simulink model "Three_Phase_180_VSI"  (R2023b)
settings: Solver=VariableStepAuto  StartTime=0.0  StopTime=0.1  RelTol=1e-3
libraries: spsDiodeLib x6, spsIGBTLib x6, spsVoltageMeasurementLib x6, spsSeriesRLCBranchLib x3, spsDCVoltageSourceLib x2, spspowerguiLib x1
settings Model: Creator=prita  LastModifiedBy=KULDIP
settings DebuggingCC: UnconnectedInputMsg=warning  UnconnectedOutputMsg=warning  UnconnectedLineMsg=warning
settings ModelReferenceCC: EnableRefExpFcnMdlSchedulingChecks=on
settings RTWCC: DLArmComputeVersion=19.05

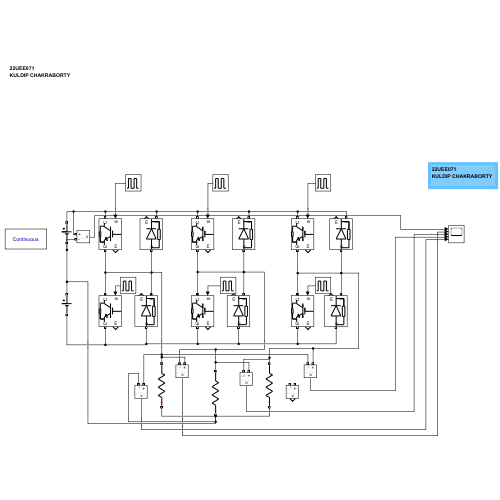
[thumbnail: Simulink's stored preview of the top-level diagram]
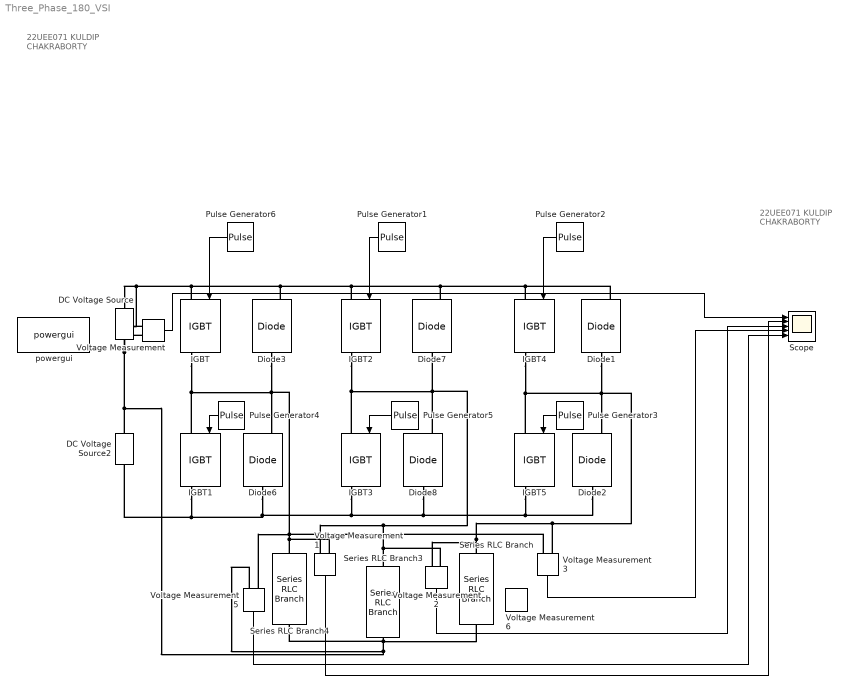
== system Three_Phase_180_VSI ==
  note: 22UEE071
      | KULDIP CHAKRABORTY
  note: 22UEE071
      | KULDIP CHAKRABORTY
  DC Voltage Source : spsDCVoltageSourceLib/DC Voltage Source  Amplitude=25  Measurements=None
  DC Voltage Source2 : spsDCVoltageSourceLib/DC Voltage Source  Amplitude=25  Measurements=None
  Diode{1..3,6..8} (6 alike) : spsDiodeLib/Diode  Ron=0.001  Lon=0  Vf=0.8  IC=0  UseSnubber=0  Rs=500  Cs=250e-9  Measurements=on
  IGBT{,1..5} (6 alike) : spsIGBTLib/IGBT  Ron=0.001  Lon=0  Vf=0  Tf=1e-6  Tt=2e-6  IC=0  Rs=1e5  Cs=inf  Measurements=on
  Pulse Generator1 : DiscretePulseGenerator  PulseType=Time based  Period=0.02  PulseWidth=50  PhaseDelay=(0.02/360)*120
  Pulse Generator2 : DiscretePulseGenerator  PulseType=Time based  Period=0.02  PulseWidth=50  PhaseDelay=(0.02/360)*240
  Pulse Generator3 : DiscretePulseGenerator  PulseType=Time based  Period=0.02  PulseWidth=50  PhaseDelay=(0.02/360)*420
  Pulse Generator4 : DiscretePulseGenerator  PulseType=Time based  Period=0.02  PulseWidth=50  PhaseDelay=(0.02/360)*180
  Pulse Generator5 : DiscretePulseGenerator  PulseType=Time based  Period=0.02  PulseWidth=50  PhaseDelay=(0.02/360)*300
  Pulse Generator6 : DiscretePulseGenerator  PulseType=Time based  Period=0.02  PulseWidth=50
  Scope : Scope  NumInputPorts=5
  Series RLC Branch : spsSeriesRLCBranchLib/Series RLC Branch  LConnTagsString=__new0  RConnTagsString=__new0  BranchType=R  Resistance=1  Inductance=1e-3  SetiL0=off  InitialCurrent=0  Capacitance=1e-6  Setx0=off  InitialVoltage=0  Measurements=None
  Series RLC Branch3 : spsSeriesRLCBranchLib/Series RLC Branch  LConnTagsString=__new0  RConnTagsString=__new0  BranchType=R  Resistance=1  Inductance=1e-3  SetiL0=off  InitialCurrent=0  Capacitance=1e-6  Setx0=off  InitialVoltage=0  Measurements=None
  Series RLC Branch4 : spsSeriesRLCBranchLib/Series RLC Branch  LConnTagsString=__new0  RConnTagsString=__new0  BranchType=R  Resistance=1  Inductance=1e-3  SetiL0=off  InitialCurrent=0  Capacitance=1e-6  Setx0=off  InitialVoltage=0  Measurements=None
  Voltage Measurement{,1..3,5..6} (6 alike) : spsVoltageMeasurementLib/Voltage Measurement  PhasorSimulation=off  OutputType=Complex  PSBequivalent=0
  powergui : spspowerguiLib/powergui  Priority=1  SimulationMode=Continuous  SampleTime=50e-6  frequency=60  Iterations=50  frequencyindice=0  Pbase=100e6  ErrMax=1e-4  UnitsV=kV  UnitsW=MW  buscounter=0  FunctionMessages=off  echomessages=off  EnableUseOfTLC=off  CurrentSourceSwitches=off  DisableSnubberDevices=off  DisableRonSwitches=off  DisableVfSwitches=off  DisplayEquations=off  AutomaticDiscreteSolvers=off  SolverType=Tustin/Backward Euler (TBE)  Interpol=off  ExternalGateDelay=off  methode=off  Ts=100  x0status=blocks  SPID=on  SwTol=0  HookPort=off  NonlinearTolerance=1e-4  nMaxIteration=100  ContinueOnMaxIteration=off  RestoreLinks=warning  ResistiveCurrentMeasurement=off  Frange=[0:2:500]  Ylog=off  Xlog=on  ShowGrid=off  save=off  variable=ZData  structure=0  ZoomFFT=off  StartTime=0.0  cycles=1  DisplayStyle=1  fundamental=60  FreqAxis=off  MaxFrequency=1000  frequencyindicesteady=1  RmsSteady=1  display=off
  wires:
  Voltage Measurement/1 -> Scope/1
  Pulse Generator6/1 -> IGBT/1
  Pulse Generator1/1 -> IGBT2/1
  Pulse Generator2/1 -> IGBT4/1
  Pulse Generator3/1 -> IGBT5/1
  Pulse Generator4/1 -> IGBT1/1
  Pulse Generator5/1 -> IGBT3/1
  Voltage Measurement1/1 -> Scope/2
  Voltage Measurement2/1 -> Scope/3
  Voltage Measurement3/1 -> Scope/4
  Voltage Measurement5/1 -> Scope/5
  connections:
  IGBT/LConn1 -- Diode1/RConn1 -- IGBT4/LConn1 -- Diode7/RConn1 -- IGBT2/LConn1 -- Diode3/RConn1 -- Voltage Measurement/LConn1 -- DC Voltage Source/RConn1
  IGBT1/RConn1 -- Diode2/LConn1 -- IGBT5/RConn1 -- Diode8/LConn1 -- IGBT3/RConn1 -- Diode6/LConn1 -- DC Voltage Source2/LConn1
  Voltage Measurement/LConn2 -- DC Voltage Source/LConn1 -- DC Voltage Source2/RConn1 -- Voltage Measurement5/LConn2 -- Series RLC Branch/LConn1 -- Series RLC Branch4/LConn1 -- Series RLC Branch3/LConn1
  Diode3/LConn1 -- Voltage Measurement5/LConn1 -- Voltage Measurement3/LConn2 -- Series RLC Branch4/RConn1 -- Voltage Measurement1/LConn1 -- IGBT1/LConn1 -- IGBT/RConn1 -- Diode6/RConn1
  Diode8/RConn1 -- IGBT2/RConn1 -- IGBT3/LConn1 -- Voltage Measurement2/LConn1 -- Series RLC Branch3/RConn1 -- Voltage Measurement1/LConn2 -- Diode7/LConn1
  Diode1/LConn1 -- Voltage Measurement2/LConn2 -- Series RLC Branch/RConn1 -- Voltage Measurement3/LConn1 -- IGBT5/LConn1 -- IGBT4/RConn1 -- Diode2/RConn1
